simulink model "estimator_discreized"  (R2017a)
settings: Solver=VariableStepAuto  StartTime=0.0  StopTime=40  RelTol=1e-3
values from neighbouring files (symbols this model uses):
  B = [b -b;-b b]    [OBS_CONT.m]    (also in OBS_CONT_MORE_STIFF.m)
  Kc = [-0.26139 0.041515 0.65538 1.1604]    [OBS_CONT.m]    (also in OBS_CONT_MORE_STIFF.m = place(F,G,p_cont))
undefined symbols (not defined in the file or in its folder): A, A_c, B_c, C, C_c, V, V_c
settings Model: Creator=ASUS  LastModifiedBy=ASUS

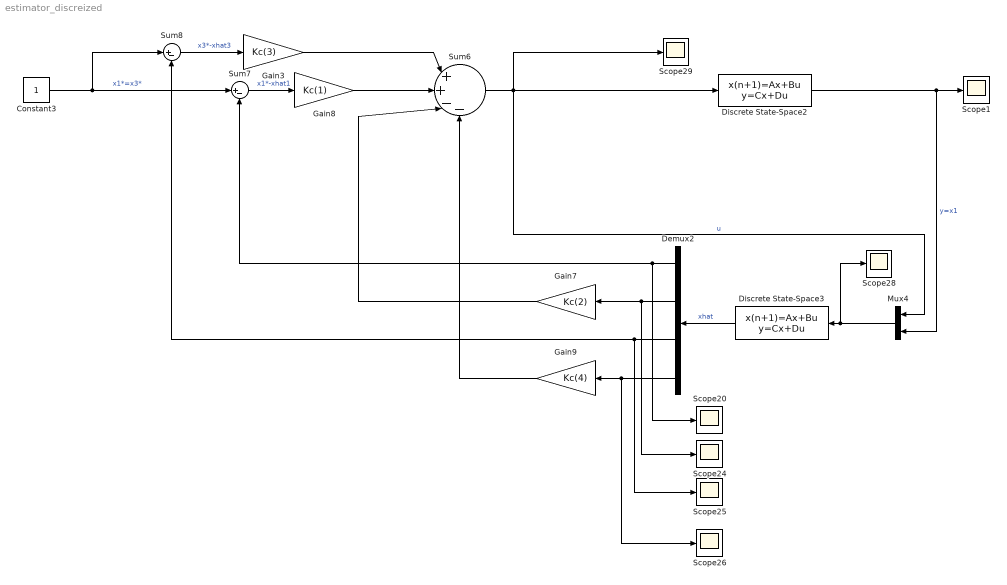
== system estimator_discreized ==
  Constant3 : Constant
  Demux2 : Demux
  Discrete State-Space2 : DiscreteStateSpace  A=A  B=B  C=C  D=V  SampleTime=0.005
  Discrete State-Space3 : DiscreteStateSpace  A=A_c  B=B_c  C=C_c  D=V_c  SampleTime=0.005
  Gain3 : Gain  Gain=Kc(3)
  Gain7 : Gain  Gain=Kc(2)
  Gain8 : Gain  Gain=Kc(1)
  Gain9 : Gain  Gain=Kc(4)
  Mux4 : Mux  Inputs=2
  Scope{1,20,24..26,28..29} (7 alike) : Scope
  Sum6 : Sum  Inputs=|++--
  Sum7 : Sum  Inputs=|+-
  Sum8 : Sum  Inputs=|+-
  wires:
  Sum6/1 -> Mux4/1, Discrete State-Space2/1, Scope29/1  "u"
  Mux4/1 -> Scope28/1, Discrete State-Space3/1
  Discrete State-Space3/1 -> Demux2/1  "xhat"
  Constant3/1 -> Sum8/1, Sum7/1  "x1*=x3*"
  Gain8/1 -> Sum6/2
  Sum7/1 -> Gain8/1  "x1*-xhat1"
  Gain3/1 -> Sum6/1
  Demux2/4 -> Scope26/1, Gain9/1
  Discrete State-Space2/1 -> Scope1/1, Mux4/2  "y=x1"
  Gain9/1 -> Sum6/4
  Demux2/3 -> Scope25/1, Sum8/2
  Demux2/2 -> Scope24/1, Gain7/1
  Gain7/1 -> Sum6/3
  Sum8/1 -> Gain3/1  "x3*-xhat3"
  Demux2/1 -> Scope20/1, Sum7/2
